simulink model "frt_MINPUT"  (R2012b)
settings: Solver=FixedStepDiscrete  SolverMode=SingleTasking  StartTime=0.0  StopTime=15000  RelTol=1e-3
undefined symbols (not defined in the file or in its folder): Down, Up
libraries: xbsIndex_r4 x3656, xps_library x3, casper_library_delays x2, simulink x1
(part 7 of 25)

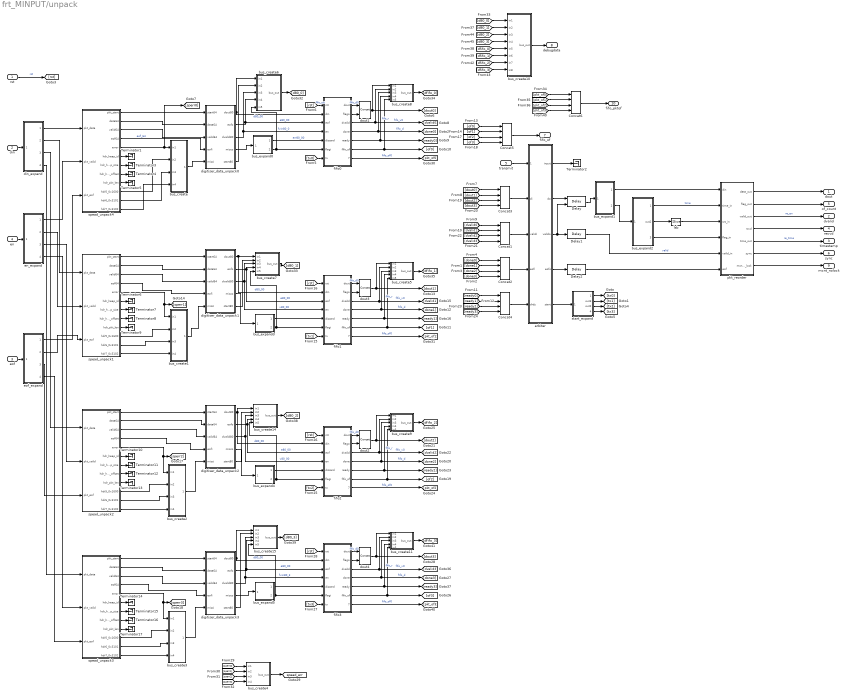
== system frt_MINPUT/unpack ==
  rst : Inport
  din : Inport  Port=2
  eof : Inport  Port=3
  en : Inport  Port=4
  transmit : Inport  Port=5
  Concat{1..6} (6 alike) : xbsIndex_r4/Concat  num_inputs=4  dbl_ovrd=off  block_type=concat
  Delay : xbsIndex_r4/Delay  rst=off  infoeditControl=Selection of Reset will increase slice count due to use of real FFs and instead of SRLs  en=on  latency=1  dbl_ovrd=off  reg_retiming=on  block_type=delay
  Delay1 : xbsIndex_r4/Delay  rst=off  infoeditControl=Selection of Reset will increase slice count due to use of real FFs and instead of SRLs  en=off  latency=1  dbl_ovrd=off  reg_retiming=on  block_type=delay
  Delay2 : xbsIndex_r4/Delay  rst=off  infoeditControl=Selection of Reset will increase slice count due to use of real FFs and instead of SRLs  en=off  latency=1  dbl_ovrd=off  reg_retiming=on  block_type=delay
  Terminator{1..17} (17 alike) : Terminator
  arbiter : Subsystem  mask{n_inputs=4, n_bits_input=160 + n_bits_timestamp + n_bits_source + n_bits_of_count, mux_latency=1, preempt=1, n_bits_block_size=n_bits_packet_size-1, n_cycles_preempt=6}
      mask prompts: n_inputs "number of inputs"; n_bits_input "input bit widths"; mux_latency "mux latency"; preempt "preempt start of next block"; n_bits_block_size "data block size (2^?)"; n_cycles_preempt "clock cycles to preempt at"
      mask init:
      | set_param([gcb, '/eofi_mux'], ...
      |     'n_bits', 'ones(1, n_inputs)', ...
      |     'mux_latency', 'mux_latency', ...
      |     'cmplx', 'off', 'misc', 'off');
      | set_param([gcb, '/di_mux'], ...
      |     'n_bits', 'repmat(n_bits_input, 1, n_inputs)', ...
      |     'mux_latency', 'mux_latency', ...
      |     'cmplx', 'off', 'misc', 'off');
      | set_param([gcb, '/validi_mux'], ...
      |     'n_bits', 'ones(1, n_inputs)', ...
      |     'mux_latency', 'mux_latency', ...
      |     'cmplx', 'off', 'misc', 'off');
      | set_param([gcb, '/busy_edge_rep'], ...
      |     'replication', 'n_inputs', ...
      |     'misc', 'off');
  bus_create : Subsystem  AncestorBlock=casper_library_flow_control/bus_create  mask(bus_create){inputNum=4}
      mask prompts: inputNum "Number of inputs:"
      mask init:
      | bus_create_init(gcb,...
      |     'inputNum', inputNum);
  bus_create1 : Subsystem  AncestorBlock=casper_library_flow_control/bus_create  mask(bus_create){inputNum=4}
      mask prompts: inputNum "Number of inputs:"
      mask init:
      | bus_create_init(gcb,...
      |     'inputNum', inputNum);
  bus_create10 : Subsystem  AncestorBlock=casper_library_flow_control/bus_create  mask(bus_create){inputNum=8}
      mask prompts: inputNum "Number of inputs:"
      mask init:
      | bus_create_init(gcb,...
      |     'inputNum', inputNum);
  bus_create11 : Subsystem  AncestorBlock=casper_library_flow_control/bus_create  mask(bus_create){inputNum=5}
      mask prompts: inputNum "Number of inputs:"
      mask init:
      | bus_create_init(gcb,...
      |     'inputNum', inputNum);
  bus_create14 : Subsystem  AncestorBlock=casper_library_flow_control/bus_create  mask(bus_create){inputNum=5}
      mask prompts: inputNum "Number of inputs:"
      mask init:
      | bus_create_init(gcb,...
      |     'inputNum', inputNum);
  bus_create15 : Subsystem  AncestorBlock=casper_library_flow_control/bus_create  mask(bus_create){inputNum=5}
      mask prompts: inputNum "Number of inputs:"
      mask init:
      | bus_create_init(gcb,...
      |     'inputNum', inputNum);
  bus_create2 : Subsystem  AncestorBlock=casper_library_flow_control/bus_create  mask(bus_create){inputNum=4}
      mask prompts: inputNum "Number of inputs:"
      mask init:
      | bus_create_init(gcb,...
      |     'inputNum', inputNum);
  bus_create3 : Subsystem  AncestorBlock=casper_library_flow_control/bus_create  mask(bus_create){inputNum=4}
      mask prompts: inputNum "Number of inputs:"
      mask init:
      | bus_create_init(gcb,...
      |     'inputNum', inputNum);
  bus_create4 : Subsystem  AncestorBlock=casper_library_flow_control/bus_create  mask(bus_create){inputNum=4}
      mask prompts: inputNum "Number of inputs:"
      mask init:
      | bus_create_init(gcb,...
      |     'inputNum', inputNum);
  bus_create5 : Subsystem  AncestorBlock=casper_library_flow_control/bus_create  mask(bus_create){inputNum=5}
      mask prompts: inputNum "Number of inputs:"
      mask init:
      | bus_create_init(gcb,...
      |     'inputNum', inputNum);
  bus_create6 : Subsystem  AncestorBlock=casper_library_flow_control/bus_create  mask(bus_create){inputNum=5}
      mask prompts: inputNum "Number of inputs:"
      mask init:
      | bus_create_init(gcb,...
      |     'inputNum', inputNum);
  bus_create7 : Subsystem  AncestorBlock=casper_library_flow_control/bus_create  mask(bus_create){inputNum=5}
      mask prompts: inputNum "Number of inputs:"
      mask init:
      | bus_create_init(gcb,...
      |     'inputNum', inputNum);
  bus_create8 : Subsystem  AncestorBlock=casper_library_flow_control/bus_create  mask(bus_create){inputNum=5}
      mask prompts: inputNum "Number of inputs:"
      mask init:
      | bus_create_init(gcb,...
      |     'inputNum', inputNum);
  bus_create9 : Subsystem  AncestorBlock=casper_library_flow_control/bus_create  mask(bus_create){inputNum=5}
      mask prompts: inputNum "Number of inputs:"
      mask init:
      | bus_create_init(gcb,...
      |     'inputNum', inputNum);
  bus_expand0 : Subsystem  AncestorBlock=casper_library_flow_control/bus_expand  mask(bus_expand){mode=divisions of arbitrary size, outputNum=1, outputWidth=[1, sum([n_bits_timestamp, n_bits_source, n_bits_of_count])], outputBinaryPt=[0 0], outputArithmeticType=[2 0], show_format=on, outputToWorkspace=off, variablePrefix=out, outputToModelAsWell=on}
      mask prompts: outputNum "Number of outputs:"; outputWidth "Output width [msb ... lsb]:"; outputBinaryPt "Output binary point position [msb ... lsb]:"; outputArithmeticType "Output arithmetic type (ufix=0, fix=1, bool=2) [msb ... lsb]:"; show_format "Print format string?"; outputToWorkspace "Output to workspace?"; variablePrefix "Variable name prefix:"; outputToModelAsWell "Output to model as well?"
      mask help:
      | Expands a 'bus' made using a bus_create or Xilinx
      | concat block.
      | The input will be divided into the specified number
      | of outputs with the specified arithmetic types.
      | Divisions are made from most significant bit.
      mask init: same as frt_MINPUT/bus_expand10
      settings: AttributesFormatString=2 outputs: b,uf144.0,
      mask TypeOptions mode: divisions of equal size | divisions of arbitrary size
      mask Callback mode: bus_expand_callback();
      mask Callback outputWidth: bus_expand_callback();
      mask Callback outputToWorkspace: bus_expand_callback();
  bus_expand1 : Subsystem  AncestorBlock=casper_library_flow_control/bus_expand  mask(bus_expand){mode=divisions of arbitrary size, outputNum=1, outputWidth=[160, sum([n_bits_timestamp, n_bits_source, n_bits_of_count])], outputBinaryPt=[0 0], outputArithmeticType=[0 0], show_format=off, outputToWorkspace=off, variablePrefix=out, outputToModelAsWell=on}
      mask prompts: outputNum "Number of outputs:"; outputWidth "Output width [msb ... lsb]:"; outputBinaryPt "Output binary point position [msb ... lsb]:"; outputArithmeticType "Output arithmetic type (ufix=0, fix=1, bool=2) [msb ... lsb]:"; show_format "Print format string?"; outputToWorkspace "Output to workspace?"; variablePrefix "Variable name prefix:"; outputToModelAsWell "Output to model as well?"
      mask help:
      | Expands a 'bus' made using a bus_create or Xilinx
      | concat block.
      | The input will be divided into the specified number
      | of outputs with the specified arithmetic types.
      | Divisions are made from most significant bit.
      mask init: same as frt_MINPUT/bus_expand10
      settings: AttributesFormatString=2 outputs
      mask TypeOptions mode: divisions of equal size | divisions of arbitrary size
      mask Callback mode: bus_expand_callback();
      mask Callback outputWidth: bus_expand_callback();
      mask Callback outputToWorkspace: bus_expand_callback();
  bus_expand2 : Subsystem  AncestorBlock=casper_library_flow_control/bus_expand  mask(bus_expand){mode=divisions of arbitrary size, outputNum=1, outputWidth=[n_bits_timestamp, n_bits_source, n_bits_of_count], outputBinaryPt=[0 0 0], outputArithmeticType=[0 0 0], show_format=off, outputToWorkspace=off, variablePrefix=out, outputToModelAsWell=on}
      mask prompts: outputNum "Number of outputs:"; outputWidth "Output width [msb ... lsb]:"; outputBinaryPt "Output binary point position [msb ... lsb]:"; outputArithmeticType "Output arithmetic type (ufix=0, fix=1, bool=2) [msb ... lsb]:"; show_format "Print format string?"; outputToWorkspace "Output to workspace?"; variablePrefix "Variable name prefix:"; outputToModelAsWell "Output to model as well?"
      mask help:
      | Expands a 'bus' made using a bus_create or Xilinx
      | concat block.
      | The input will be divided into the specified number
      | of outputs with the specified arithmetic types.
      | Divisions are made from most significant bit.
      mask init: same as frt_MINPUT/bus_expand10
      settings: AttributesFormatString=3 outputs
      mask TypeOptions mode: divisions of equal size | divisions of arbitrary size
      mask Callback mode: bus_expand_callback();
      mask Callback outputWidth: bus_expand_callback();
      mask Callback outputToWorkspace: bus_expand_callback();
  bus_expand3 : Subsystem  AncestorBlock=casper_library_flow_control/bus_expand  mask(bus_expand){mode=divisions of arbitrary size, outputNum=1, outputWidth=[1, sum([n_bits_timestamp, n_bits_source, n_bits_of_count])], outputBinaryPt=[0 0], outputArithmeticType=[2 0], show_format=off, outputToWorkspace=off, variablePrefix=out, outputToModelAsWell=on}
      mask prompts: outputNum "Number of outputs:"; outputWidth "Output width [msb ... lsb]:"; outputBinaryPt "Output binary point position [msb ... lsb]:"; outputArithmeticType "Output arithmetic type (ufix=0, fix=1, bool=2) [msb ... lsb]:"; show_format "Print format string?"; outputToWorkspace "Output to workspace?"; variablePrefix "Variable name prefix:"; outputToModelAsWell "Output to model as well?"
      mask help:
      | Expands a 'bus' made using a bus_create or Xilinx
      | concat block.
      | The input will be divided into the specified number
      | of outputs with the specified arithmetic types.
      | Divisions are made from most significant bit.
      mask init: same as frt_MINPUT/bus_expand10
      settings: AttributesFormatString=2 outputs
      mask TypeOptions mode: divisions of equal size | divisions of arbitrary size
      mask Callback mode: bus_expand_callback();
      mask Callback outputWidth: bus_expand_callback();
      mask Callback outputToWorkspace: bus_expand_callback();
  bus_expand4 : Subsystem  AncestorBlock=casper_library_flow_control/bus_expand  mask(bus_expand){mode=divisions of arbitrary size, outputNum=1, outputWidth=[1, sum([n_bits_timestamp, n_bits_source, n_bits_of_count])], outputBinaryPt=[0 0], outputArithmeticType=[2 0], show_format=off, outputToWorkspace=off, variablePrefix=out, outputToModelAsWell=on}
      mask prompts: outputNum "Number of outputs:"; outputWidth "Output width [msb ... lsb]:"; outputBinaryPt "Output binary point position [msb ... lsb]:"; outputArithmeticType "Output arithmetic type (ufix=0, fix=1, bool=2) [msb ... lsb]:"; show_format "Print format string?"; outputToWorkspace "Output to workspace?"; variablePrefix "Variable name prefix:"; outputToModelAsWell "Output to model as well?"
      mask help:
      | Expands a 'bus' made using a bus_create or Xilinx
      | concat block.
      | The input will be divided into the specified number
      | of outputs with the specified arithmetic types.
      | Divisions are made from most significant bit.
      mask init: same as frt_MINPUT/bus_expand10
      settings: AttributesFormatString=2 outputs
      mask TypeOptions mode: divisions of equal size | divisions of arbitrary size
      mask Callback mode: bus_expand_callback();
      mask Callback outputWidth: bus_expand_callback();
      mask Callback outputToWorkspace: bus_expand_callback();
  bus_expand5 : Subsystem  AncestorBlock=casper_library_flow_control/bus_expand  mask(bus_expand){mode=divisions of arbitrary size, outputNum=1, outputWidth=[1, sum([n_bits_timestamp, n_bits_source, n_bits_of_count])], outputBinaryPt=[0 0], outputArithmeticType=[2 0], show_format=off, outputToWorkspace=off, variablePrefix=out, outputToModelAsWell=on}
      mask prompts: outputNum "Number of outputs:"; outputWidth "Output width [msb ... lsb]:"; outputBinaryPt "Output binary point position [msb ... lsb]:"; outputArithmeticType "Output arithmetic type (ufix=0, fix=1, bool=2) [msb ... lsb]:"; show_format "Print format string?"; outputToWorkspace "Output to workspace?"; variablePrefix "Variable name prefix:"; outputToModelAsWell "Output to model as well?"
      mask help:
      | Expands a 'bus' made using a bus_create or Xilinx
      | concat block.
      | The input will be divided into the specified number
      | of outputs with the specified arithmetic types.
      | Divisions are made from most significant bit.
      mask init: same as frt_MINPUT/bus_expand10
      settings: AttributesFormatString=2 outputs
      mask TypeOptions mode: divisions of equal size | divisions of arbitrary size
      mask Callback mode: bus_expand_callback();
      mask Callback outputWidth: bus_expand_callback();
      mask Callback outputToWorkspace: bus_expand_callback();
  digitiser_data_unpack0 : Subsystem
  digitiser_data_unpack1 : Subsystem
  digitiser_data_unpack2 : Subsystem
  digitiser_data_unpack3 : Subsystem
  din_expand : Subsystem  AncestorBlock=casper_library_flow_control/bus_expand  mask(bus_expand){mode=divisions of equal size, outputNum=4, outputWidth=64, outputBinaryPt=0, outputArithmeticType=0, show_format=off, outputToWorkspace=off, variablePrefix=out, outputToModelAsWell=on}
      mask prompts: outputNum "Number of outputs:"; outputWidth "Output width:"; outputBinaryPt "Output binary point position:"; outputArithmeticType "Output arithmetic type (ufix=0, fix=1, bool=2):"; show_format "Print format string?"; outputToWorkspace "Output to workspace?"; variablePrefix "Variable name prefix:"; outputToModelAsWell "Output to model as well?"
      mask help:
      | Expands a 'bus' made using a bus_create or Xilinx
      | concat block.
      | The input will be divided into the specified number
      | of outputs with the specified arithmetic types.
      | Divisions are made from most significant bit.
      mask init: same as frt_MINPUT/bus_expand10
      settings: AttributesFormatString=4 outputs
      mask TypeOptions mode: divisions of equal size | divisions of arbitrary size
      mask Callback mode: bus_expand_callback();
      mask Callback outputWidth: bus_expand_callback();
      mask Callback outputToWorkspace: bus_expand_callback();
  dout{1..4} (4 alike) : xbsIndex_r4/Concat  num_inputs=2  dbl_ovrd=off  block_type=concat
  en_expand : Subsystem  AncestorBlock=casper_library_flow_control/bus_expand  mask(bus_expand){mode=divisions of equal size, outputNum=4, outputWidth=1, outputBinaryPt=0, outputArithmeticType=2, show_format=off, outputToWorkspace=off, variablePrefix=out, outputToModelAsWell=on}
      mask prompts: outputNum "Number of outputs:"; outputWidth "Output width:"; outputBinaryPt "Output binary point position:"; outputArithmeticType "Output arithmetic type (ufix=0, fix=1, bool=2):"; show_format "Print format string?"; outputToWorkspace "Output to workspace?"; variablePrefix "Variable name prefix:"; outputToModelAsWell "Output to model as well?"
      mask help:
      | Expands a 'bus' made using a bus_create or Xilinx
      | concat block.
      | The input will be divided into the specified number
      | of outputs with the specified arithmetic types.
      | Divisions are made from most significant bit.
      mask init: same as frt_MINPUT/bus_expand10
      settings: AttributesFormatString=4 outputs
      mask TypeOptions mode: divisions of equal size | divisions of arbitrary size
      mask Callback mode: bus_expand_callback();
      mask Callback outputWidth: bus_expand_callback();
      mask Callback outputToWorkspace: bus_expand_callback();
  eof_expand : Subsystem  AncestorBlock=casper_library_flow_control/bus_expand  mask(bus_expand){mode=divisions of equal size, outputNum=4, outputWidth=1, outputBinaryPt=0, outputArithmeticType=2, show_format=off, outputToWorkspace=off, variablePrefix=out, outputToModelAsWell=on}
      mask prompts: outputNum "Number of outputs:"; outputWidth "Output width:"; outputBinaryPt "Output binary point position:"; outputArithmeticType "Output arithmetic type (ufix=0, fix=1, bool=2):"; show_format "Print format string?"; outputToWorkspace "Output to workspace?"; variablePrefix "Variable name prefix:"; outputToModelAsWell "Output to model as well?"
      mask help:
      | Expands a 'bus' made using a bus_create or Xilinx
      | concat block.
      | The input will be divided into the specified number
      | of outputs with the specified arithmetic types.
      | Divisions are made from most significant bit.
      mask init: same as frt_MINPUT/bus_expand10
      settings: AttributesFormatString=4 outputs
      mask TypeOptions mode: divisions of equal size | divisions of arbitrary size
      mask Callback mode: bus_expand_callback();
      mask Callback outputWidth: bus_expand_callback();
      mask Callback outputToWorkspace: bus_expand_callback();
  fifo0 : Subsystem  mask{n_bits_din=80, n_bits_depth=2, n_bits_flag=sum([n_bits_timestamp, n_bits_source, n_bits_of_count]), scale_factor_bits=1, input_word_count_bits=n_bits_packet_size, bram_latency=bram_latency}
      mask prompts: n_bits_din "input data bit width"; n_bits_depth "max buffer depth (2^? packets)"; n_bits_flag "flag bit width"; scale_factor_bits "output width scale factor (2^?)"; input_word_count_bits "max input word count (2^?)"; bram_latency "BRAM latency"
  fifo1 : Subsystem  mask{n_bits_din=80, n_bits_depth=2, n_bits_flag=sum([n_bits_timestamp, n_bits_source, n_bits_of_count]), scale_factor_bits=1, input_word_count_bits=n_bits_packet_size, bram_latency=bram_latency}
      mask prompts: n_bits_din "input data bit width"; n_bits_depth "max buffer depth (2^? packets)"; n_bits_flag "flag bit width"; scale_factor_bits "output width scale factor (2^?)"; input_word_count_bits "max input word count (2^?)"; bram_latency "BRAM latency"
  fifo2 : Subsystem  mask{n_bits_din=80, n_bits_depth=2, n_bits_flag=sum([n_bits_timestamp, n_bits_source, n_bits_of_count]), scale_factor_bits=1, input_word_count_bits=n_bits_packet_size, bram_latency=bram_latency}
      mask prompts: n_bits_din "input data bit width"; n_bits_depth "max buffer depth (2^? packets)"; n_bits_flag "flag bit width"; scale_factor_bits "output width scale factor (2^?)"; input_word_count_bits "max input word count (2^?)"; bram_latency "BRAM latency"
  fifo3 : Subsystem  mask{n_bits_din=80, n_bits_depth=2, n_bits_flag=sum([n_bits_timestamp, n_bits_source, n_bits_of_count]), scale_factor_bits=1, input_word_count_bits=n_bits_packet_size, bram_latency=bram_latency}
      mask prompts: n_bits_din "input data bit width"; n_bits_depth "max buffer depth (2^? packets)"; n_bits_flag "flag bit width"; scale_factor_bits "output width scale factor (2^?)"; input_word_count_bits "max input word count (2^?)"; bram_latency "BRAM latency"
  lsb : xbsIndex_r4/Slice  nbits=1  boolean_output=off  mode=Lower Bit Location + Width  bit1=0  base1=MSB of Input  bit0=0  base0=LSB of Input  dbl_ovrd=off  block_type=slice
  pkt_reorder : Subsystem  mask{window_bits=n_bits_buffer, window_size_bits=n_bits_packet_size - 1, n_bits_din=80, n_bits_flag=n_bits_of_count, n_bits_timestamp=n_bits_timestamp}
      mask prompts: window_bits "Number of Windows to Buffer (2^?)"; window_size_bits "Window size (2^?)"; n_bits_din "Data bit width in"; n_bits_flag "Flag bit width in"; n_bits_timestamp "Timestamp bit width"
      mask init:
      | fmtstr = sprintf('Buffer space: 2^%i words', window_bits+window_size_bits);
      | set_param(gcb, 'AttributesFormatString', fmtstr);
      settings: AttributesFormatString=Buffer space: 2^11 words
  spead_unpack1 : Subsystem  Tag=casper:spead_unpack  AncestorBlock=casper_library_communications/spead_unpack  mask(spead_unpack_mask){max_pkt_len_bits=10, header_ids=[5632 12545 12546], spead_msw=64, spead_lsw=48, spead_version=4, combine_errors=on}
      mask prompts: max_pkt_len_bits "Max pkt length, 2^? 64-bit words"; header_ids "SPEAD header IDs (decimal)"; spead_msw "SPEAD Flavour (MSw)"; spead_lsw "SPEAD Flavour (LSw)"; spead_version "SPEAD version"; combine_errors "Combine error flags"
      mask help: This block receives a 64-bit-word stream that contains a SPEAD stream. It checks the SPEAD headers are being correctly received. It presents the user with all headers on the first valid cycle of data along with a flag to indicate a header or packet-length error.
      mask init:
      | spead_unpack_init(gcb)
  spead_unpack2 : Subsystem  Tag=casper:spead_unpack  AncestorBlock=casper_library_communications/spead_unpack  mask(spead_unpack_mask){max_pkt_len_bits=10, header_ids=[5632 12545 12546], spead_msw=64, spead_lsw=48, spead_version=4, combine_errors=on}
      mask prompts: max_pkt_len_bits "Max pkt length, 2^? 64-bit words"; header_ids "SPEAD header IDs (decimal)"; spead_msw "SPEAD Flavour (MSw)"; spead_lsw "SPEAD Flavour (LSw)"; spead_version "SPEAD version"; combine_errors "Combine error flags"
      mask help: This block receives a 64-bit-word stream that contains a SPEAD stream. It checks the SPEAD headers are being correctly received. It presents the user with all headers on the first valid cycle of data along with a flag to indicate a header or packet-length error.
      mask init:
      | spead_unpack_init(gcb)
  spead_unpack3 : Subsystem  Tag=casper:spead_unpack  AncestorBlock=casper_library_communications/spead_unpack  mask(spead_unpack_mask){max_pkt_len_bits=10, header_ids=[5632 12545 12546], spead_msw=64, spead_lsw=48, spead_version=4, combine_errors=on}
      mask prompts: max_pkt_len_bits "Max pkt length, 2^? 64-bit words"; header_ids "SPEAD header IDs (decimal)"; spead_msw "SPEAD Flavour (MSw)"; spead_lsw "SPEAD Flavour (LSw)"; spead_version "SPEAD version"; combine_errors "Combine error flags"
      mask help: This block receives a 64-bit-word stream that contains a SPEAD stream. It checks the SPEAD headers are being correctly received. It presents the user with all headers on the first valid cycle of data along with a flag to indicate a header or packet-length error.
      mask init:
      | spead_unpack_init(gcb)
  spead_unpack4 : Subsystem  Tag=casper:spead_unpack  AncestorBlock=casper_library_communications/spead_unpack  mask(spead_unpack_mask){max_pkt_len_bits=10, header_ids=[5632 12545 12546], spead_msw=64, spead_lsw=48, spead_version=4, combine_errors=on}
      mask prompts: max_pkt_len_bits "Max pkt length, 2^? 64-bit words"; header_ids "SPEAD header IDs (decimal)"; spead_msw "SPEAD Flavour (MSw)"; spead_lsw "SPEAD Flavour (LSw)"; spead_version "SPEAD version"; combine_errors "Combine error flags"
      mask help: This block receives a 64-bit-word stream that contains a SPEAD stream. It checks the SPEAD headers are being correctly received. It presents the user with all headers on the first valid cycle of data along with a flag to indicate a header or packet-length error.
      mask init:
      | spead_unpack_init(gcb)
  start_expand : Subsystem  AncestorBlock=casper_library_flow_control/bus_expand  mask(bus_expand){mode=divisions of equal size, outputNum=4, outputWidth=1, outputBinaryPt=0, outputArithmeticType=2, show_format=off, outputToWorkspace=off, variablePrefix=out, outputToModelAsWell=on}
      mask prompts: outputNum "Number of outputs:"; outputWidth "Output width:"; outputBinaryPt "Output binary point position:"; outputArithmeticType "Output arithmetic type (ufix=0, fix=1, bool=2):"; show_format "Print format string?"; outputToWorkspace "Output to workspace?"; variablePrefix "Variable name prefix:"; outputToModelAsWell "Output to model as well?"
      mask help:
      | Expands a 'bus' made using a bus_create or Xilinx
      | concat block.
      | The input will be divided into the specified number
      | of outputs with the specified arithmetic types.
      | Divisions are made from most significant bit.
      mask init: same as frt_MINPUT/bus_expand10
      settings: AttributesFormatString=4 outputs
      mask TypeOptions mode: divisions of equal size | divisions of arbitrary size
      mask Callback mode: bus_expand_callback();
      mask Callback outputWidth: bus_expand_callback();
      mask Callback outputToWorkspace: bus_expand_callback();
  dout : Outport
  dvalid : Outport  Port=2
  timestamp : Outport  Port=3
  recvd : Outport  Port=4
  of_count : Outport  Port=5
  sync : Outport  Port=6
  fifo_of : Outport  Port=7
  debugdata : Outport  Port=8
  mcnt_nolock : Outport  Port=9
  fifo_pktof : Outport  Port=10
  tag scope: spead_err=global
  wires:
  [dfifo_0] -> bus_create10/5(in5)
  [dfifo_3] -> bus_create10/8(in8)
  [dfifo_2] -> bus_create10/7(in7)
  [dfifo_1] -> bus_create10/6(in6)
  [d80_3] -> bus_create10/4(in4)
  [d80_2] -> bus_create10/3(in3)
  [d80_1] -> bus_create10/2(in2)
  [d80_0] -> bus_create10/1(in1)
  digitiser_data_unpack3/5(start80) -> bus_create15/2(in2)
  digitiser_data_unpack2/5(start80) -> bus_create14/2(in2)
  bus_create15/1(bus_out) -> [d80_3]
  bus_create14/1(bus_out) -> [d80_2]
  [tx1] -> fifo1/7(tx)
  [tx0] -> fifo0/7(tx)
  pkt_reorder/7(mcnt_no_lock) -> mcnt_nolock/1
  pkt_reorder/6(sync) -> sync/1
  pkt_reorder/5(time_out) -> timestamp/1  "re_time"
  pkt_reorder/4(rcvd) -> recvd/1
  pkt_reorder/3(valid_out) -> dvalid/1  "re_en"
  pkt_reorder/2(flag_out) -> of_count/1
  pkt_reorder/1(data_out) -> dout/1
  digitiser_data_unpack1/5(start80) -> bus_create7/2(in2)
  bus_create7/1(bus_out) -> [d80_1]
  digitiser_data_unpack0/5(start80) -> bus_create6/2(in2)
  spead_unpack4/3(valid64) -> digitiser_data_unpack0/3(valid64)
  spead_unpack4/10(hdr5_0x1600) -> bus_create/2(in2)
  bus_create10/1(bus_out) -> debugdata/1
  bus_create8/1(bus_out) -> [dfifo_0]
  bus_create6/1(bus_out) -> [d80_0]
  fifo0/4(done) -> [done0], bus_create8/3(in3)  "fifo_d"
  dout1/1 -> bus_create8/1(in1), [dout0]
  fifo0/3(dvalid) -> [dvalid0], bus_create8/2(in2)  "fifo_v0"
  fifo0/5(ready) -> [ready0], bus_create8/4(in4)  "fifo_r"
  arbiter/5(start) -> start_expand/1(bus_in)
  Concat4/1 -> arbiter/5(drdy)
  Concat2/1 -> arbiter/4(eofi)
  Concat3/1 -> arbiter/2(di)
  Concat1/1 -> arbiter/3(validi)
  transmit/1 -> arbiter/1(transmit)
  start_expand/1(msb_out4) -> [tx0]
  start_expand/2(out3) -> [tx1]
  start_expand/3(out2) -> [tx2]
  start_expand/4(lsb_out1) -> [tx3]
  [done0] -> Concat2/1
  [done3] -> Concat2/4
  [done1] -> Concat2/2
  [done2] -> Concat2/3
  [dout0] -> Concat3/1
  [dout1] -> Concat3/2
  [dvalid0] -> Concat1/1
  [dvalid1] -> Concat1/2
  [ready0] -> Concat4/1
  [ready1] -> Concat4/2
  Concat5/1 -> fifo_of/1
  [dout2] -> Concat3/3
  [dout3] -> Concat3/4
  [dvalid2] -> Concat1/3
  [dvalid3] -> Concat1/4
  [ready2] -> Concat4/3
  [ready3] -> Concat4/4
  arbiter/1(input) -> Terminator2/1
  [of0] -> Concat5/1
  [of1] -> Concat5/2
  [of2] -> Concat5/3
  [of3] -> Concat5/4
  rst/1 -> [rst]  "rst"
  [rst] -> fifo0/1(rst)  "fifo_rst"
  din/1 -> din_expand/1(bus_in)
  en/1 -> en_expand/1(bus_in)
  eof/1 -> eof_expand/1(bus_in)
  digitiser_data_unpack0/1(dout80) -> fifo0/2(din), bus_create6/1(in1)  "d80_00"
  digitiser_data_unpack0/4(misco) -> bus_expand0/1(bus_in)
  digitiser_data_unpack0/2(eofo) -> fifo0/3(eof), bus_create6/4(in4)  "e80_00"
  digitiser_data_unpack0/3(dvalid80) -> fifo0/4(en), bus_create6/3(in3)  "fvin80_0"
  bus_expand1/1(msb_out2) -> pkt_reorder/1(din)
  bus_expand1/2(lsb_out1) -> bus_expand2/1(bus_in)
  bus_expand2/1(msb_out3) -> pkt_reorder/2(time_in)  "time"
  bus_expand2/3(lsb_out1) -> pkt_reorder/4(flag_in)
  spead_unpack4/1(pkt_start) -> digitiser_data_unpack0/1(start64)
  spead_unpack1/1(pkt_start) -> digitiser_data_unpack1/1(start64)
  spead_unpack2/1(pkt_start) -> digitiser_data_unpack2/1(start64)
  spead_unpack3/1(pkt_start) -> digitiser_data_unpack3/1(start64)
  spead_unpack4/2(data64) -> digitiser_data_unpack0/2(data64)
  spead_unpack4/4(eof64) -> digitiser_data_unpack0/4(eofi)  "eof_64"
  bus_create/1(bus_out) -> digitiser_data_unpack0/5(misci)
  bus_expand0/1(msb_out2) -> fifo0/5(discard)  "err80_00"
  bus_expand0/2(lsb_out1) -> fifo0/6(flagi), bus_create6/5(in5)
  spead_unpack1/3(valid64) -> digitiser_data_unpack1/3(valid64)
  spead_unpack1/4(eof64) -> digitiser_data_unpack1/4(eofi)
  spead_unpack1/5(error) -> bus_create1/1(in1), [sperr1]
  spead_unpack1/10(hdr5_0x1600) -> bus_create1/2(in2)
  spead_unpack1/11(hdr6_0x3101) -> bus_create1/3(in3)
  spead_unpack1/12(hdr7_0x3102) -> bus_create1/4(in4)
  bus_create1/1(bus_out) -> digitiser_data_unpack1/5(misci)
  spead_unpack2/2(data64) -> digitiser_data_unpack2/2(data64)
  spead_unpack2/3(valid64) -> digitiser_data_unpack2/3(valid64)
  spead_unpack2/4(eof64) -> digitiser_data_unpack2/4(eofi)
  spead_unpack2/5(error) -> [sperr2], bus_create2/1(in1)
  spead_unpack2/10(hdr5_0x1600) -> bus_create2/2(in2)
  spead_unpack2/11(hdr6_0x3101) -> bus_create2/3(in3)
  spead_unpack2/12(hdr7_0x3102) -> bus_create2/4(in4)
  bus_create2/1(bus_out) -> digitiser_data_unpack2/5(misci)
  spead_unpack3/2(data64) -> digitiser_data_unpack3/2(data64)
  spead_unpack3/3(valid64) -> digitiser_data_unpack3/3(valid64)
  spead_unpack3/4(eof64) -> digitiser_data_unpack3/4(eofi)
  spead_unpack3/5(error) -> bus_create3/1(in1), [sperr3]
  spead_unpack3/10(hdr5_0x1600) -> bus_create3/2(in2)
  spead_unpack3/11(hdr6_0x3101) -> bus_create3/3(in3)
  spead_unpack3/12(hdr7_0x3102) -> bus_create3/4(in4)
  bus_create3/1(bus_out) -> digitiser_data_unpack3/5(misci)
  [rst] -> fifo1/1(rst)
  digitiser_data_unpack1/1(dout80) -> fifo1/2(din), bus_create7/1(in1)  "d80_00"
  digitiser_data_unpack1/4(misco) -> bus_expand3/1(bus_in)
  digitiser_data_unpack1/2(eofo) -> fifo1/3(eof), bus_create7/4(in4)  "e80_00"
  digitiser_data_unpack1/3(dvalid80) -> fifo1/4(en), bus_create7/3(in3)  "v80_00"
  bus_expand3/1(msb_out2) -> fifo1/5(discard)
  bus_expand3/2(lsb_out1) -> fifo1/6(flagi), bus_create7/5(in5)
  [tx2] -> fifo2/7(tx)
  [rst] -> fifo2/1(rst)
  digitiser_data_unpack2/1(dout80) -> fifo2/2(din), bus_create14/1(in1)  "d80_00"
  digitiser_data_unpack2/4(misco) -> bus_expand4/1(bus_in)
  digitiser_data_unpack2/2(eofo) -> fifo2/3(eof), bus_create14/4(in4)  "e80_00"
  digitiser_data_unpack2/3(dvalid80) -> fifo2/4(en), bus_create14/3(in3)  "v80_00"
  bus_expand4/1(msb_out2) -> fifo2/5(discard)
  bus_expand4/2(lsb_out1) -> fifo2/6(flagi), bus_create14/5(in5)
  fifo0/1(dout) -> dout1/1  "fifo_d0"
  fifo0/2(flago) -> dout1/2
  [tx3] -> fifo3/7(tx)
  [rst] -> fifo3/1(rst)
  digitiser_data_unpack3/1(dout80) -> fifo3/2(din), bus_create15/1(in1)  "d80_00"
  digitiser_data_unpack3/4(misco) -> bus_expand5/1(bus_in)
  digitiser_data_unpack3/2(eofo) -> fifo3/3(eof), bus_create15/4(in4)  "e80_00"
  digitiser_data_unpack3/3(dvalid80) -> fifo3/4(en), bus_create15/3(in3)  "fvin80_3"
  bus_expand5/1(msb_out2) -> fifo3/5(discard)
  bus_expand5/2(lsb_out1) -> fifo3/6(flagi), bus_create15/5(in5)
  bus_expand2/2(out2) -> lsb/1
  lsb/1 -> pkt_reorder/3(src_in)
  spead_unpack4/5(error) -> bus_create/1(in1), [sperr0]
  spead_unpack4/11(hdr6_0x3101) -> bus_create/3(in3)
  spead_unpack4/12(hdr7_0x3102) -> bus_create/4(in4)
  arbiter/2(do) -> Delay/1
  arbiter/3(valido) -> Delay1/1, Delay/2
  arbiter/4(eofo) -> Delay2/1
  Delay/1 -> bus_expand1/1(bus_in)
  Delay1/1 -> pkt_reorder/5(valid_in)  "valid"
  Delay2/1 -> pkt_reorder/6(eof)
  [sperr0] -> bus_create4/1(in1)
  [sperr1] -> bus_create4/2(in2)
  [sperr2] -> bus_create4/3(in3)
  [sperr3] -> bus_create4/4(in4)
  bus_create4/1(bus_out) -> [spead_err]
  fifo0/6(fifo_of) -> bus_create8/5(in5), [of0]
  fifo0/7(packet_of) -> [pkt_of0]  "fifo_of0"
  bus_create5/1(bus_out) -> [dfifo_1]
  fifo1/4(done) -> [done1], bus_create5/3(in3)  "fifo_d"
  dout3/1 -> [dout1], bus_create5/1(in1)
  fifo1/3(dvalid) -> [dvalid1], bus_create5/2(in2)  "fifo_v0"
  fifo1/5(ready) -> [ready1], bus_create5/4(in4)  "fifo_r"
  fifo1/1(dout) -> dout3/1  "fifo_d0"
  fifo1/2(flago) -> dout3/2
  fifo1/6(fifo_of) -> [of1], bus_create5/5(in5)
  fifo1/7(packet_of) -> [pkt_of1]  "fifo_of0"
  bus_create9/1(bus_out) -> [dfifo_2]
  fifo2/4(done) -> bus_create9/3(in3), [done2]  "fifo_d"
  dout2/1 -> bus_create9/1(in1), [dout2]
  fifo2/3(dvalid) -> bus_create9/2(in2), [dvalid2]  "fifo_v0"
  fifo2/5(ready) -> bus_create9/4(in4), [ready2]  "fifo_r"
  fifo2/1(dout) -> dout2/1  "fifo_d0"
  fifo2/2(flago) -> dout2/2
  fifo2/6(fifo_of) -> bus_create9/5(in5), [of2]
  fifo2/7(packet_of) -> [pkt_of2]  "fifo_of0"
  bus_create11/1(bus_out) -> [dfifo_3]
  fifo3/4(done) -> [done3], bus_create11/3(in3)  "fifo_d"
  dout4/1 -> [dout3], bus_create11/1(in1)
  fifo3/3(dvalid) -> [dvalid3], bus_create11/2(in2)  "fifo_v0"
  fifo3/5(ready) -> [ready3], bus_create11/4(in4)  "fifo_r"
  fifo3/1(dout) -> dout4/1  "fifo_d0"
  fifo3/2(flago) -> dout4/2
  fifo3/6(fifo_of) -> [of3], bus_create11/5(in5)
  fifo3/7(packet_of) -> [pkt_of3]  "fifo_of0"
  Concat6/1 -> fifo_pktof/1
  [pkt_of0] -> Concat6/1
  [pkt_of1] -> Concat6/2
  [pkt_of2] -> Concat6/3
  [pkt_of3] -> Concat6/4
  spead_unpack4/6(hdr_heap_id) -> Terminator1/1
  spead_unpack4/7(hdr_heap_size) -> Terminator3/1
  spead_unpack4/8(hdr_heap_offset) -> Terminator4/1
  spead_unpack4/9(hdr_pkt_len) -> Terminator5/1
  spead_unpack1/6(hdr_heap_id) -> Terminator6/1
  spead_unpack1/7(hdr_heap_size) -> Terminator7/1
  spead_unpack1/8(hdr_heap_offset) -> Terminator8/1
  spead_unpack1/9(hdr_pkt_len) -> Terminator9/1
  spead_unpack2/6(hdr_heap_id) -> Terminator10/1
  spead_unpack2/7(hdr_heap_size) -> Terminator11/1
  spead_unpack2/8(hdr_heap_offset) -> Terminator12/1
  spead_unpack2/9(hdr_pkt_len) -> Terminator13/1
  spead_unpack3/6(hdr_heap_id) -> Terminator14/1
  spead_unpack3/7(hdr_heap_size) -> Terminator15/1
  spead_unpack3/8(hdr_heap_offset) -> Terminator16/1
  spead_unpack3/9(hdr_pkt_len) -> Terminator17/1
  din_expand/1(msb_out4) -> spead_unpack4/1(pkt_data)
  en_expand/1(msb_out4) -> spead_unpack4/2(pkt_valid)
  eof_expand/1(msb_out4) -> spead_unpack4/3(pkt_eof)
  en_expand/2(out3) -> spead_unpack1/2(pkt_valid)
  din_expand/2(out3) -> spead_unpack1/1(pkt_data)
  eof_expand/2(out3) -> spead_unpack1/3(pkt_eof)
  din_expand/3(out2) -> spead_unpack2/1(pkt_data)
  din_expand/4(lsb_out1) -> spead_unpack3/1(pkt_data)
  en_expand/3(out2) -> spead_unpack2/2(pkt_valid)
  eof_expand/3(out2) -> spead_unpack2/3(pkt_eof)
  en_expand/4(lsb_out1) -> spead_unpack3/2(pkt_valid)
  eof_expand/4(lsb_out1) -> spead_unpack3/3(pkt_eof)
  spead_unpack1/2(data64) -> digitiser_data_unpack1/2(data64)

== system frt_MINPUT/ct/bus_expand ==
  bus_in : Inport
  reinterpret{1..4} (4 alike) : xbsIndex_r4/Reinterpret  force_arith_type=on  arith_type=Unsigned  force_bin_pt=on  bin_pt=0  block_type=reinterpret
  slice1 : xbsIndex_r4/Slice  nbits=64  boolean_output=off  mode=Upper Bit Location + Width  bit1=-192  base1=MSB of Input  bit0=0  base0=LSB of Input  dbl_ovrd=off  block_type=slice
  slice2 : xbsIndex_r4/Slice  nbits=64  boolean_output=off  mode=Upper Bit Location + Width  bit1=-128  base1=MSB of Input  bit0=0  base0=LSB of Input  dbl_ovrd=off  block_type=slice
  slice3 : xbsIndex_r4/Slice  nbits=64  boolean_output=off  mode=Upper Bit Location + Width  bit1=-64  base1=MSB of Input  bit0=0  base0=LSB of Input  dbl_ovrd=off  block_type=slice
  slice4 : xbsIndex_r4/Slice  nbits=64  boolean_output=off  mode=Upper Bit Location + Width  bit1=0  base1=MSB of Input  bit0=0  base0=LSB of Input  dbl_ovrd=off  block_type=slice
  msb_out4 : Outport
  out3 : Outport  Port=2
  out2 : Outport  Port=3
  lsb_out1 : Outport  Port=4
  wires:
  reinterpret1/1 -> lsb_out1/1
  slice1/1 -> reinterpret1/1
  reinterpret2/1 -> out2/1
  slice2/1 -> reinterpret2/1
  reinterpret3/1 -> out3/1
  slice3/1 -> reinterpret3/1
  reinterpret4/1 -> msb_out4/1
  slice4/1 -> reinterpret4/1
  bus_in/1 -> slice1/1, slice2/1, slice3/1, slice4/1
